simulink model "seesaw_mod_lin_non_lin"  (R2013a)
settings: Solver=ode3  StartTime=0.0  StopTime=30  RelTol=1e-3
values from neighbouring files (symbols this model uses):
  A = [0 mf*g*h/Jconst 0 -mf*g/Jconst;1 0 0 0;0 -g 0 0;0 0 1 0]    [seesaw_ini.m]
  B = [1/Jconst;0;0;0]    [seesaw_ini.m]
  C = [0 0 0 1]    [seesaw_ini.m]
  c = eye(4)    [seesaw_ini.m]
  D = [0;0;0;0]    [seesaw_ini.m]
  g = 9.81    [seesaw_ini.m]
  H = HT.'    [seesaw_ini.m]
  h = 0.1    [seesaw_ini.m]
  Hd = Htd.'    [seesaw_ini.m]
  Jconst = Jb + mf*h*h    (= 0.501)    [seesaw_ini.m]
  k2 = K2-p*C    [seesaw_ini.m]
  K2 = K_hat(1:4)    [seesaw_ini.m]
  mf = 0.1    [seesaw_ini.m]
  p = 1/(C*((B*k-A)^-1)*B)    [seesaw_ini.m]
  PI = K_hat(5)    [seesaw_ini.m]
  Ts = 1/8000    (= 0.000125)    [seesaw_ini.m]
undefined symbols (not defined in the file or in its folder): Ad, Bd
settings Model: Creator=Xone  LastModifiedBy=ALI

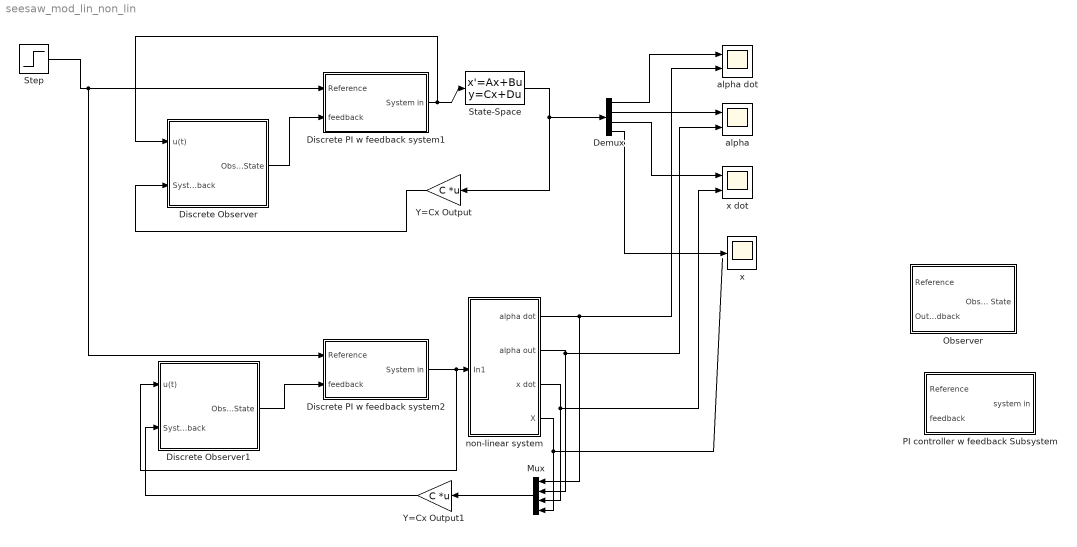
== system seesaw_mod_lin_non_lin ==
  Demux : Demux
  Discrete Observer : Subsystem
  Discrete Observer1 : Subsystem
  Discrete PI w feedback system1 : Subsystem
  Discrete PI w feedback system2 : Subsystem
  Mux : Mux
  Observer : Subsystem
  PI controller w feedback Subsystem : Subsystem
  State-Space : StateSpace  A=A  B=B  C=c  D=D  X0=[0;0;0;0.05]
  Step : Step  SampleTime=0
  Y=Cx Output : Gain  Gain=C  Multiplication=Matrix(K*u)
  Y=Cx Output1 : Gain  Gain=C  Multiplication=Matrix(K*u)
  alpha : Scope  NumInputPorts=2
      settings: YMin=-5~-5  YMax=5~5  SaveName=alphalin
  alpha dot : Scope  NumInputPorts=2
      settings: TimeRange=10  YMin=-5~-5  YMax=5~5  SaveName=adotlin
  non-linear system : Subsystem
  x : Scope
      settings: SaveName=xlin
  x dot : Scope  NumInputPorts=2
      settings: YMin=-5~-5  YMax=5~5  SaveName=xdotlin
  wires:
  State-Space/1 -> Y=Cx Output/1, Demux/1
  Demux/1 -> alpha dot/1
  Demux/2 -> alpha/1
  Demux/3 -> x dot/1
  Demux/4 -> x/1
  Y=Cx Output/1 -> Discrete Observer/2(System Feedback)
  Mux/1 -> Y=Cx Output1/1
  Step/1 -> Discrete PI w feedback system1/1(Reference), Discrete PI w feedback system2/1(Reference)
  Discrete Observer/1(Observed State) -> Discrete PI w feedback system1/2(" feedback")
  non-linear system/1(alpha dot) -> alpha dot/2, Mux/1
  non-linear system/2(alpha out) -> alpha/2, Mux/2
  non-linear system/3(x dot) -> x dot/2, Mux/3
  non-linear system/4("X ") -> Mux/4
  Y=Cx Output1/1 -> Discrete Observer1/2(System Feedback)
  Discrete PI w feedback system1/1(System in) -> Discrete Observer/1(u(t)), State-Space/1
  Discrete PI w feedback system2/1(System in) -> Discrete Observer1/1(u(t)), non-linear system/1(In1)
  Discrete Observer1/1(Observed State) -> Discrete PI w feedback system2/2(" feedback")

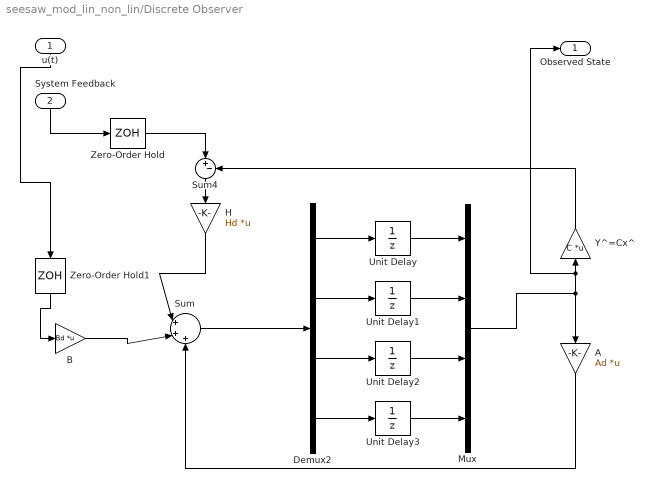
== system seesaw_mod_lin_non_lin/Discrete Observer ==
  u(t) : Inport
  System Feedback : Inport  Port=2
  "A " : Gain  Gain=Ad  Multiplication=Matrix(K*u)
  B : Gain  Gain=Bd  Multiplication=Matrix(K*u) (u vector)
  Demux2 : Demux
  H : Gain  Gain=Hd  Multiplication=Matrix(K*u) (u vector)
  Mux : Mux
  Sum : Sum  Inputs=|+++
  Sum4 : Sum  Inputs=|+-
  Unit Delay{,1..3} (4 alike) : UnitDelay  SampleTime=-1
  Y^=Cx^ : Gain  Gain=C  Multiplication=Matrix(K*u)
  Zero-Order Hold : ZeroOrderHold  SampleTime=Ts
  Zero-Order Hold1 : ZeroOrderHold  SampleTime=Ts
  Observed State : Outport
  wires:
  B/1 -> Sum/2
  H/1 -> Sum/1
  Sum/1 -> Demux2/1
  Mux/1 -> Y^=Cx^/1, Observed State/1, "A "/1
  "A "/1 -> Sum/3
  Zero-Order Hold1/1 -> B/1
  Unit Delay1/1 -> Mux/2
  Unit Delay/1 -> Mux/1
  Zero-Order Hold/1 -> Sum4/1
  Y^=Cx^/1 -> Sum4/2
  Demux2/4 -> Unit Delay3/1
  Demux2/3 -> Unit Delay2/1
  Demux2/2 -> Unit Delay1/1
  Demux2/1 -> Unit Delay/1
  System Feedback/1 -> Zero-Order Hold/1
  u(t)/1 -> Zero-Order Hold1/1
  Unit Delay3/1 -> Mux/4
  Unit Delay2/1 -> Mux/3
  Sum4/1 -> H/1

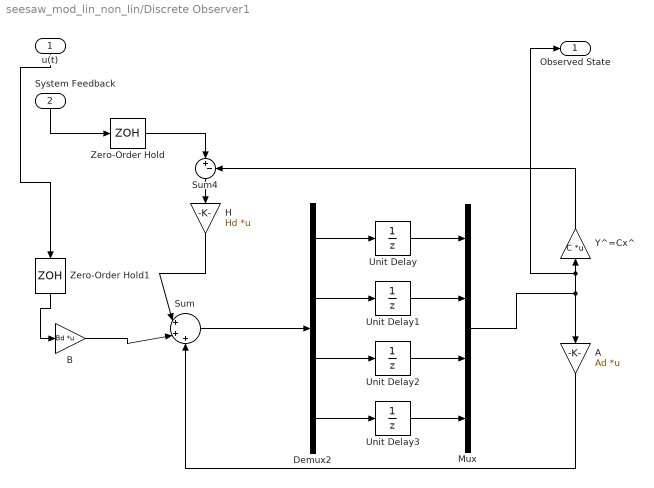
== system seesaw_mod_lin_non_lin/Discrete Observer1 ==
  u(t) : Inport
  System Feedback : Inport  Port=2
  "A " : Gain  Gain=Ad  Multiplication=Matrix(K*u)
  B : Gain  Gain=Bd  Multiplication=Matrix(K*u) (u vector)
  Demux2 : Demux
  H : Gain  Gain=Hd  Multiplication=Matrix(K*u) (u vector)
  Mux : Mux
  Sum : Sum  Inputs=|+++
  Sum4 : Sum  Inputs=|+-
  Unit Delay{,1..3} (4 alike) : UnitDelay  SampleTime=-1
  Y^=Cx^ : Gain  Gain=C  Multiplication=Matrix(K*u)
  Zero-Order Hold : ZeroOrderHold  SampleTime=Ts
  Zero-Order Hold1 : ZeroOrderHold  SampleTime=Ts
  Observed State : Outport
  wires:
  Sum4/1 -> H/1
  Unit Delay2/1 -> Mux/3
  Unit Delay3/1 -> Mux/4
  u(t)/1 -> Zero-Order Hold1/1
  System Feedback/1 -> Zero-Order Hold/1
  Demux2/1 -> Unit Delay/1
  Demux2/2 -> Unit Delay1/1
  Demux2/3 -> Unit Delay2/1
  Demux2/4 -> Unit Delay3/1
  Y^=Cx^/1 -> Sum4/2
  Zero-Order Hold/1 -> Sum4/1
  Unit Delay/1 -> Mux/1
  Unit Delay1/1 -> Mux/2
  Zero-Order Hold1/1 -> B/1
  "A "/1 -> Sum/3
  Mux/1 -> "A "/1, Observed State/1, Y^=Cx^/1
  Sum/1 -> Demux2/1
  H/1 -> Sum/1
  B/1 -> Sum/2

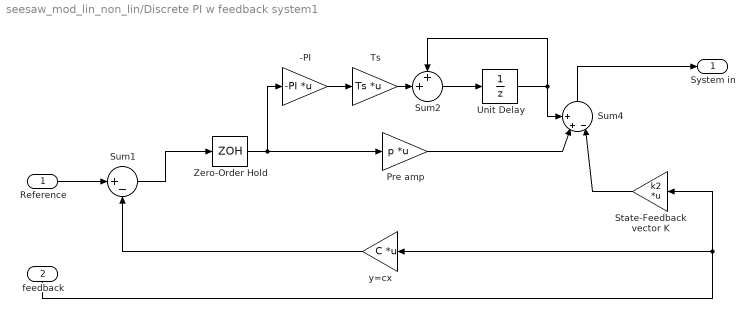
== system seesaw_mod_lin_non_lin/Discrete PI w feedback system1 ==
  Reference : Inport
  " feedback" : Inport  Port=2
  -PI : Gain  Gain=-PI  Multiplication=Matrix(K*u) (u vector)
  Pre amp : Gain  Gain=p  Multiplication=Matrix(K*u) (u vector)
  State-Feedback vector K : Gain  Gain=k2  Multiplication=Matrix(K*u) (u vector)
  Sum1 : Sum  Inputs=|+-
  Sum2 : Sum  Inputs=++|
  Sum4 : Sum  Inputs=++-|
  Ts : Gain  Gain=Ts  Multiplication=Matrix(K*u) (u vector)
  Unit Delay : UnitDelay  SampleTime=-1
  Zero-Order Hold : ZeroOrderHold  SampleTime=Ts
  y=cx : Gain  Gain=C  Multiplication=Matrix(K*u) (u vector)
  System in : Outport
  wires:
  Reference/1 -> Sum1/1
  " feedback"/1 -> y=cx/1, State-Feedback vector K/1
  State-Feedback vector K/1 -> Sum4/3
  -PI/1 -> Ts/1
  Unit Delay/1 -> Sum4/1, Sum2/1
  Ts/1 -> Sum2/2
  Sum4/1 -> System in/1
  y=cx/1 -> Sum1/2
  Sum1/1 -> Zero-Order Hold/1
  Zero-Order Hold/1 -> -PI/1, Pre amp/1
  Pre amp/1 -> Sum4/2
  Sum2/1 -> Unit Delay/1

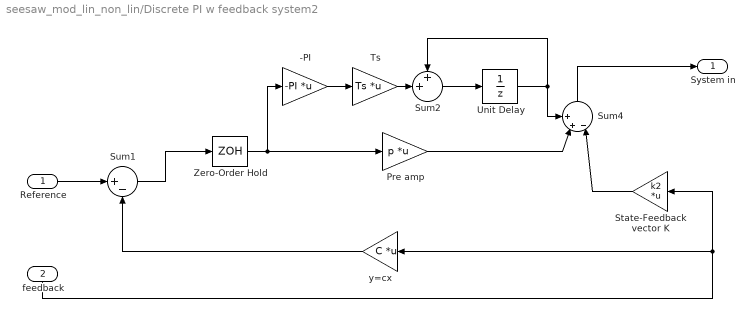
== system seesaw_mod_lin_non_lin/Discrete PI w feedback system2 ==
  Reference : Inport
  " feedback" : Inport  Port=2
  -PI : Gain  Gain=-PI  Multiplication=Matrix(K*u) (u vector)
  Pre amp : Gain  Gain=p  Multiplication=Matrix(K*u) (u vector)
  State-Feedback vector K : Gain  Gain=k2  Multiplication=Matrix(K*u) (u vector)
  Sum1 : Sum  Inputs=|+-
  Sum2 : Sum  Inputs=++|
  Sum4 : Sum  Inputs=++-|
  Ts : Gain  Gain=Ts  Multiplication=Matrix(K*u) (u vector)
  Unit Delay : UnitDelay  SampleTime=-1
  Zero-Order Hold : ZeroOrderHold  SampleTime=Ts
  y=cx : Gain  Gain=C  Multiplication=Matrix(K*u) (u vector)
  System in : Outport
  wires:
  Sum2/1 -> Unit Delay/1
  Pre amp/1 -> Sum4/2
  Zero-Order Hold/1 -> Pre amp/1, -PI/1
  Sum1/1 -> Zero-Order Hold/1
  y=cx/1 -> Sum1/2
  Sum4/1 -> System in/1
  Ts/1 -> Sum2/2
  Unit Delay/1 -> Sum2/1, Sum4/1
  -PI/1 -> Ts/1
  State-Feedback vector K/1 -> Sum4/3
  " feedback"/1 -> State-Feedback vector K/1, y=cx/1
  Reference/1 -> Sum1/1

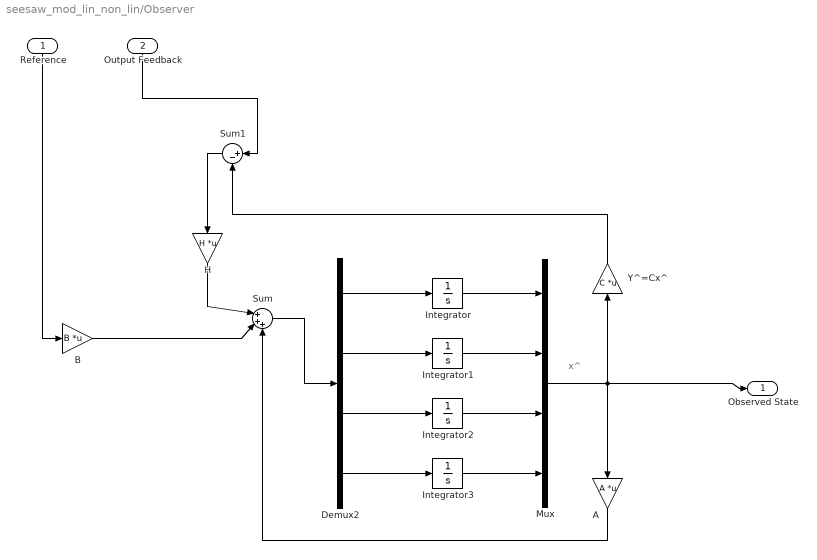
== system seesaw_mod_lin_non_lin/Observer ==
  note: x^
  Reference : Inport
  Output Feedback : Inport  Port=2
  "A " : Gain  Gain=A  Multiplication=Matrix(K*u)
  B : Gain  Gain=B  Multiplication=Matrix(K*u)
  Demux2 : Demux
  H : Gain  Gain=H  Multiplication=Matrix(K*u)
  Integrator{,1..3} (4 alike) : Integrator
  Mux : Mux
  Sum : Sum  Inputs=|+++
  Sum1 : Sum  Inputs=|+-
  Y^=Cx^ : Gain  Gain=C  Multiplication=Matrix(K*u)
  Observed State : Outport
  wires:
  Reference/1 -> B/1
  Output Feedback/1 -> Sum1/1
  Y^=Cx^/1 -> Sum1/2
  Sum1/1 -> H/1
  Sum/1 -> Demux2/1
  "A "/1 -> Sum/3
  H/1 -> Sum/1
  B/1 -> Sum/2
  Integrator2/1 -> Mux/3
  Integrator1/1 -> Mux/2
  Integrator/1 -> Mux/1
  Mux/1 -> Y^=Cx^/1, Observed State/1, "A "/1
  Integrator3/1 -> Mux/4
  Demux2/4 -> Integrator3/1
  Demux2/3 -> Integrator2/1
  Demux2/2 -> Integrator1/1
  Demux2/1 -> Integrator/1

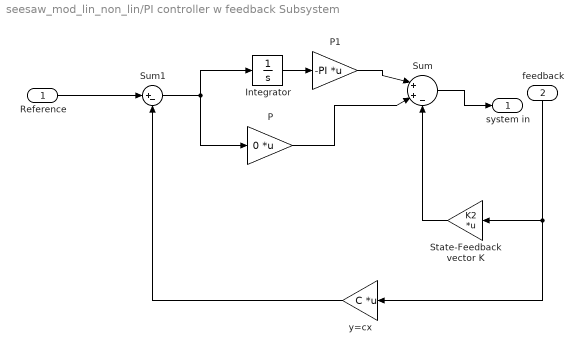
== system seesaw_mod_lin_non_lin/PI controller w feedback Subsystem ==
  Reference : Inport
  "feedback " : Inport  Port=2
  Integrator : Integrator
  P : Gain  Gain=0  Multiplication=Matrix(K*u) (u vector)
  P1 : Gain  Gain=-PI  Multiplication=Matrix(K*u) (u vector)
  State-Feedback vector K : Gain  Gain=K2  Multiplication=Matrix(K*u) (u vector)
  Sum : Sum  Inputs=|++-
  Sum1 : Sum  Inputs=|+-
  y=cx : Gain  Gain=C  Multiplication=Matrix(K*u) (u vector)
  system in : Outport
  wires:
  Sum1/1 -> Integrator/1, P/1
  P/1 -> Sum/2
  State-Feedback vector K/1 -> Sum/3
  Integrator/1 -> P1/1
  y=cx/1 -> Sum1/2
  P1/1 -> Sum/1
  Sum/1 -> system in/1
  Reference/1 -> Sum1/1
  "feedback "/1 -> State-Feedback vector K/1, y=cx/1

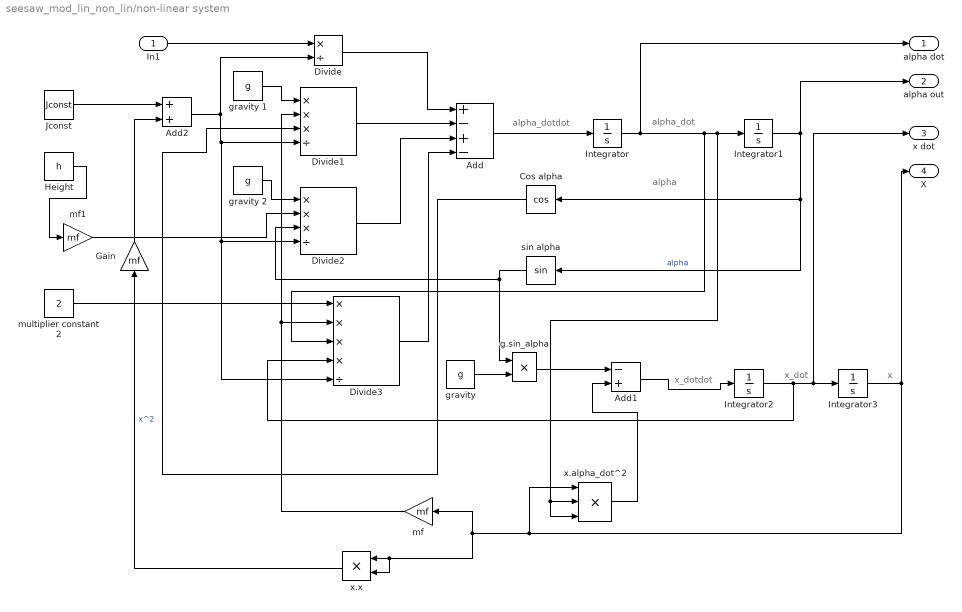
== system seesaw_mod_lin_non_lin/non-linear system ==
  note: alpha
  note: alpha_dotdot
  note: alpha_dot
  note: x_dotdot
  note: x_dot
  note: x
  In1 : Inport
  Add : Sum  Inputs=+-+-
  Add1 : Sum  Inputs=-+
  Add2 : Sum
  Cos alpha : Trigonometry  Operator=cos
  Divide : Product  Inputs=*/
  Divide1 : Product  Inputs=***/
  Divide2 : Product  Inputs=***/
  Divide3 : Product  Inputs=****/
  Gain : Gain  Gain=mf
  Height : Constant  Value=h
  Integrator{,1..3} (4 alike) : Integrator
  "Jconst " : Constant  Value=Jconst
  g.sin_alpha : Product  Inputs=**
  "gravity " : Constant  Value=g
  gravity 1 : Constant  Value=g
  gravity 2 : Constant  Value=g
  mf : Gain  Gain=mf
  mf1 : Gain  Gain=mf
  multiplier constant 2 : Constant  Value=2
  sin alpha : Trigonometry
  x.alpha_dot^2 : Product  Inputs=***
  x.x : Product  Inputs=**
  alpha dot : Outport
  alpha out : Outport  Port=2
  x dot : Outport  Port=3
  "X " : Outport  Port=4
  wires:
  Add/1 -> Integrator/1
  Integrator/1 -> alpha dot/1, Divide3/3, x.alpha_dot^2/3, x.alpha_dot^2/2, Integrator1/1
  Add1/1 -> Integrator2/1
  Integrator2/1 -> Divide3/4, x dot/1, Integrator3/1
  Divide/1 -> Add/1
  Integrator3/1 -> x.alpha_dot^2/1, mf/1, x.x/1, x.x/2, "X "/1
  x.x/1 -> Gain/1  "x^2"
  "Jconst "/1 -> Add2/1
  Gain/1 -> Add2/2
  sin alpha/1 -> Divide2/3, g.sin_alpha/1
  "gravity "/1 -> g.sin_alpha/2
  x.alpha_dot^2/1 -> Add1/2
  Divide1/1 -> Add/2
  Divide2/1 -> Add/3
  Height/1 -> mf1/1
  Integrator1/1 -> alpha out/1, Cos alpha/1, sin alpha/1  "alpha"
  Divide3/1 -> Add/4
  g.sin_alpha/1 -> Add1/1
  In1/1 -> Divide/1
  Add2/1 -> Divide/2, Divide3/5, Divide2/4, Divide1/4
  Cos alpha/1 -> Divide1/3
  mf/1 -> Divide3/2, Divide1/2
  gravity 1/1 -> Divide1/1
  gravity 2/1 -> Divide2/1
  mf1/1 -> Divide2/2
  multiplier constant 2/1 -> Divide3/1
